simulink model "PlantSimulationLABControl"  (R2019a)
settings: Solver=ode4  StartTime=0.0  StopTime=inf  FixedStep=1e-4  RelTol=1e-3
undefined symbols (not defined in the file): TF15, TF15m, TF30, TF30m
libraries: simulink x4
settings Model: EnablePacing=on  Creator=jenei  LastModifiedBy=bohor

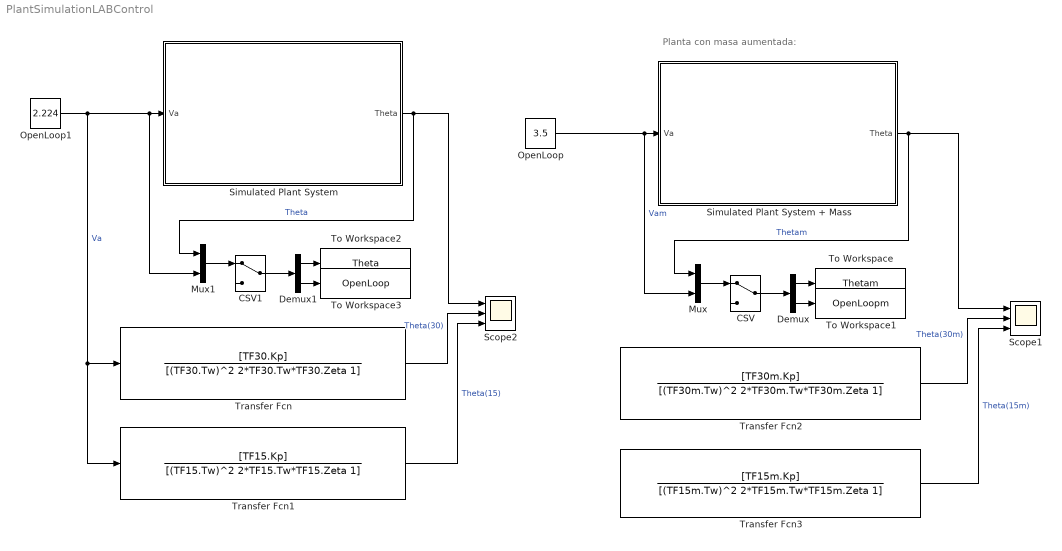
== system PlantSimulationLABControl ==
  note: Planta con masa aumentada:
  CSV : ManualSwitch
  CSV1 : ManualSwitch
  Demux : Demux  Outputs=2
  Demux1 : Demux  Outputs=2
  Mux : Mux  Inputs=2
  Mux1 : Mux  Inputs=2
  OpenLoop : Constant  Value=3.5
  OpenLoop1 : Constant  Value=2.224
  Scope1 : Scope  NumInputPorts=3
  Scope2 : Scope  NumInputPorts=3
  Simulated Plant System : Subsystem  mask{l=0, m=0, kp=0, b=0, vabar=0}
      mask init:
      | l = 0.15; % [m]
      | m = 0.15; % [kg]
      | Kp = 0.15; % [s*A/m]
      | b = 0.2; % [kg*m/s]
      | syms x
      | vabar = solve((Kp/m)*x^2-9.8*cos(deg2rad(-45)) == 0);
      | vabar = abs(double(vabar(1)));
  Simulated Plant System + Mass : Subsystem  mask{l=0, m=0, kp=0, b=0, vabar=0}
      mask init:
      | l = 0.15; % [m]
      | m = 0.4; % [kg]
      | Kp = 0.15; % [s*A/m]
      | b = 0.2; % [kg*m/s]
      | syms x
      | vabar = solve((Kp/m)*x^2-9.8*cos(deg2rad(-45)) == 0);
      | vabar = abs(double(vabar(1)));
  To Workspace : ToWorkspace  VariableName=Thetam  SampleTime=0.021
      settings: Save2DSignal=2-D array (concatenate along first dimension)
  To Workspace1 : ToWorkspace  VariableName=OpenLoopm  SampleTime=0.021
      settings: Save2DSignal=2-D array (concatenate along first dimension)
  To Workspace2 : ToWorkspace  VariableName=Theta  SampleTime=0.021
      settings: Save2DSignal=2-D array (concatenate along first dimension)
  To Workspace3 : ToWorkspace  VariableName=OpenLoop  SampleTime=0.021
      settings: Save2DSignal=2-D array (concatenate along first dimension)
  Transfer Fcn : TransferFcn  Numerator=[TF30.Kp]  Denominator=[(TF30.Tw)^2 2*TF30.Tw*TF30.Zeta 1]
  Transfer Fcn1 : TransferFcn  Numerator=[TF15.Kp]  Denominator=[(TF15.Tw)^2 2*TF15.Tw*TF15.Zeta 1]
  Transfer Fcn2 : TransferFcn  Numerator=[TF30m.Kp]  Denominator=[(TF30m.Tw)^2 2*TF30m.Tw*TF30m.Zeta 1]
  Transfer Fcn3 : TransferFcn  Numerator=[TF15m.Kp]  Denominator=[(TF15m.Tw)^2 2*TF15m.Tw*TF15m.Zeta 1]
  wires:
  OpenLoop/1 -> Mux/2, Simulated Plant System + Mass/1(Va)  "Vam"
  Simulated Plant System + Mass/1(Theta) -> Mux/1, Scope1/1  "Thetam"
  Mux/1 -> CSV/1
  CSV/1 -> Demux/1
  Demux/1 -> To Workspace/1
  Demux/2 -> To Workspace1/1
  CSV1/1 -> Demux1/1
  OpenLoop1/1 -> Transfer Fcn1/1, Transfer Fcn/1, Mux1/2, Simulated Plant System/1(Va)  "Va"
  Mux1/1 -> CSV1/1
  Simulated Plant System/1(Theta) -> Mux1/1, Scope2/1  "Theta"
  Demux1/1 -> To Workspace2/1
  Demux1/2 -> To Workspace3/1
  Transfer Fcn/1 -> Scope2/2  "Theta(30)"
  Transfer Fcn1/1 -> Scope2/3  "Theta(15)"
  Transfer Fcn2/1 -> Scope1/2  "Theta(30m)"
  Transfer Fcn3/1 -> Scope1/3  "Theta(15m)"

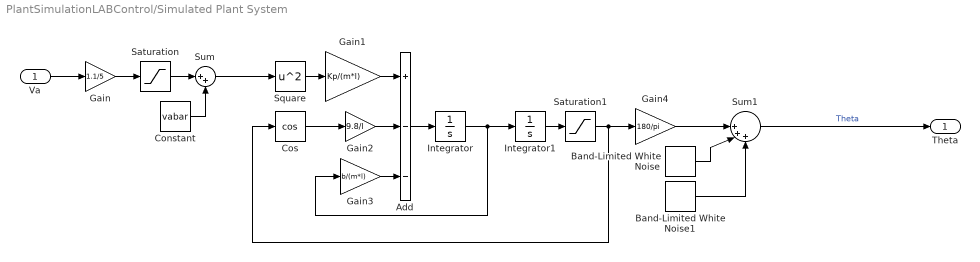
== system PlantSimulationLABControl/Simulated Plant System ==
  Va : Inport
  Add : Sum  Inputs=+--
  Band-Limited White Noise : simulink/Sources/Band-Limited White Noise  Cov=[0.00005]  Ts=0.05  seed=[23341]
  Band-Limited White Noise1 : simulink/Sources/Band-Limited White Noise  Cov=[0.01]  Ts=1  seed=[23341]
  Constant : Constant  Value=vabar
  Cos : Trigonometry  Operator=cos
  Gain : Gain  Gain=1.1/5
  Gain1 : Gain  Gain=Kp/(m*l)
  Gain2 : Gain  Gain=9.8/l
  Gain3 : Gain  Gain=b/(m*l)
  Gain4 : Gain  Gain=180/pi
  Integrator : Integrator
  Integrator1 : Integrator  InitialCondition=deg2rad(-45)
  Saturation : Saturate  UpperLimit=5  LowerLimit=0
  Saturation1 : Saturate  UpperLimit=deg2rad(90)  LowerLimit=deg2rad(-45)
  Square : Math  Operator=square  SaturateOnIntegerOverflow=on
  Sum : Sum  Inputs=|++
  Sum1 : Sum  Inputs=||+++
  Theta : Outport  VectorParamsAs1DForOutWhenUnconnected=on
  wires:
  Gain4/1 -> Sum1/1
  Integrator/1 -> Integrator1/1, Gain3/1
  Band-Limited White Noise/1 -> Sum1/2
  Add/1 -> Integrator/1
  Gain1/1 -> Add/1
  Integrator1/1 -> Saturation1/1
  Gain2/1 -> Add/2
  Square/1 -> Gain1/1
  Cos/1 -> Gain2/1
  Sum1/1 -> Theta/1  "Theta"
  Gain3/1 -> Add/3
  Band-Limited White Noise1/1 -> Sum1/3
  Va/1 -> Gain/1
  Constant/1 -> Sum/2
  Saturation/1 -> Sum/1
  Gain/1 -> Saturation/1
  Saturation1/1 -> Cos/1, Gain4/1
  Sum/1 -> Square/1

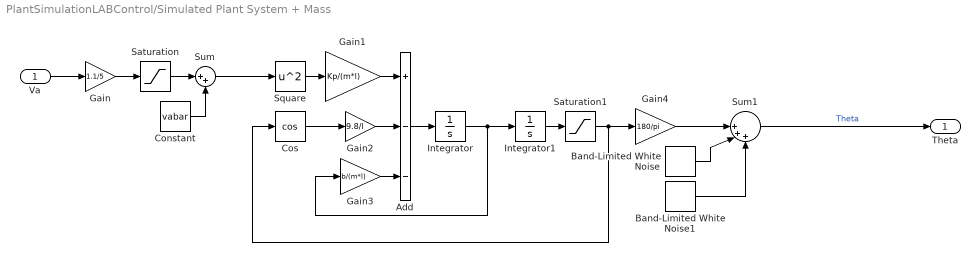
== system PlantSimulationLABControl/Simulated Plant System + Mass ==
  Va : Inport
  Add : Sum  Inputs=+--
  Band-Limited White Noise : simulink/Sources/Band-Limited White Noise  Cov=[0.00005]  Ts=0.05  seed=[23341]
  Band-Limited White Noise1 : simulink/Sources/Band-Limited White Noise  Cov=[0.01]  Ts=1  seed=[23341]
  Constant : Constant  Value=vabar
  Cos : Trigonometry  Operator=cos
  Gain : Gain  Gain=1.1/5
  Gain1 : Gain  Gain=Kp/(m*l)
  Gain2 : Gain  Gain=9.8/l
  Gain3 : Gain  Gain=b/(m*l)
  Gain4 : Gain  Gain=180/pi
  Integrator : Integrator
  Integrator1 : Integrator  InitialCondition=deg2rad(-45)
  Saturation : Saturate  UpperLimit=5  LowerLimit=0
  Saturation1 : Saturate  UpperLimit=deg2rad(90)  LowerLimit=deg2rad(-45)
  Square : Math  Operator=square  SaturateOnIntegerOverflow=on
  Sum : Sum  Inputs=|++
  Sum1 : Sum  Inputs=||+++
  Theta : Outport  VectorParamsAs1DForOutWhenUnconnected=on
  wires:
  Gain4/1 -> Sum1/1
  Integrator/1 -> Integrator1/1, Gain3/1
  Band-Limited White Noise/1 -> Sum1/2
  Add/1 -> Integrator/1
  Gain1/1 -> Add/1
  Integrator1/1 -> Saturation1/1
  Gain2/1 -> Add/2
  Square/1 -> Gain1/1
  Cos/1 -> Gain2/1
  Sum1/1 -> Theta/1  "Theta"
  Gain3/1 -> Add/3
  Band-Limited White Noise1/1 -> Sum1/3
  Va/1 -> Gain/1
  Constant/1 -> Sum/2
  Saturation/1 -> Sum/1
  Gain/1 -> Saturation/1
  Saturation1/1 -> Cos/1, Gain4/1
  Sum/1 -> Square/1
